simulink model "bao28b"  (R2014a)
settings: Solver=ode45  StartTime=0.0  StopTime=10.0  RelTol=1e-3
settings Model: Creator=Lan  LastModifiedBy=Lan

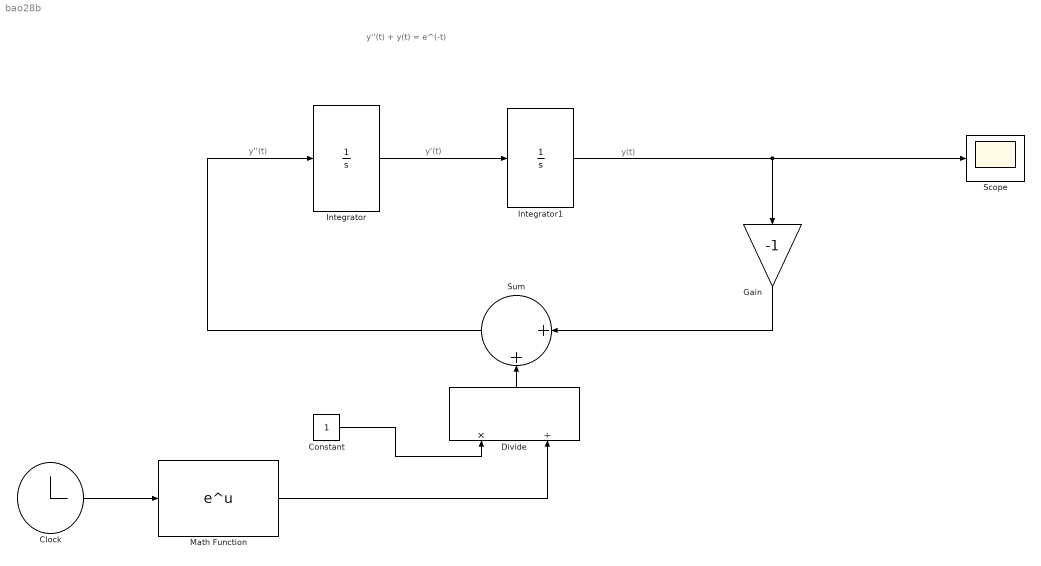
== system bao28b ==
  note: y''(t)
  note: y(t)
  note: y'(t)
  note: y''(t) + y(t) = e^(-t)
  Clock : Clock
  Constant : Constant
  Divide : Product  Inputs=*/
  Gain : Gain  Gain=-1
  Integrator : Integrator
  Integrator1 : Integrator
  Math Function : Math  SaturateOnIntegerOverflow=on
  Scope : Scope
  Sum : Sum  Inputs=|++
  wires:
  Clock/1 -> Math Function/1
  Integrator/1 -> Integrator1/1
  Integrator1/1 -> Gain/1, Scope/1
  Gain/1 -> Sum/1
  Sum/1 -> Integrator/1
  Divide/1 -> Sum/2
  Math Function/1 -> Divide/2
  Constant/1 -> Divide/1
